simulink model "antiwindup_blockDiagram"  (R2025b)
settings: Solver=FixedStepAuto  StartTime=0.0  StopTime=5.0  FixedStep=0.01  RelTol=1e-3
model workspace (MAT data in the model file):
  Kawd = 1
  Ki = 1
  Kp = 1
values from neighbouring files (symbols this model uses):
  mu1 = 2.668    [StepResponseComparison.m]
  T1 = 0.47    [StepResponseComparison.m]
  Ts = time(2) - time(1)    [AntiwindupComparison.m]    (also in StepResponseComparison.m)
settings Model: Creator=favar  LastModifiedBy=favar

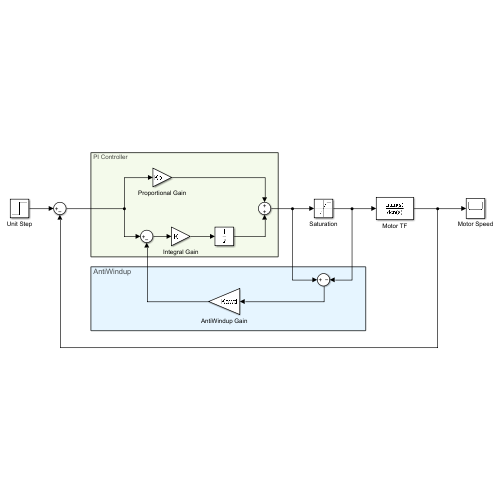
[thumbnail: Simulink's stored preview of the top-level diagram]
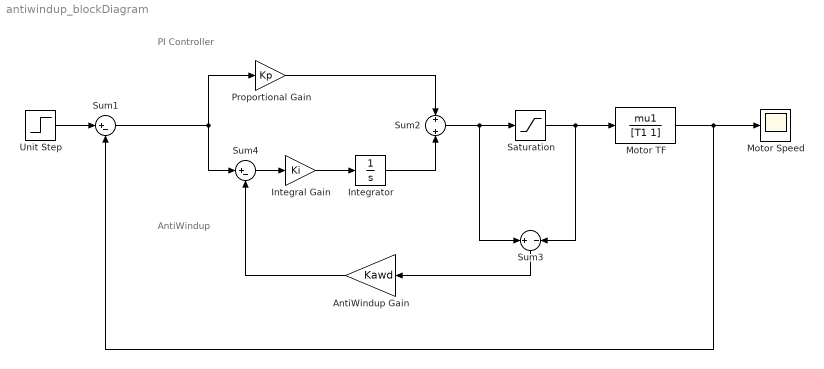
== system antiwindup_blockDiagram ==
  note: AntiWindup
  note: PI Controller
  AntiWindup Gain : Gain  Gain=Kawd
  Integral Gain : Gain  Gain=Ki
  Integrator : Integrator
  Motor Speed : Scope
  Motor TF : TransferFcn  Numerator=mu1  Denominator=[T1 1]
  Proportional Gain : Gain  Gain=Kp  RndMeth=Zero
  Saturation : Saturate
  Sum1 : Sum  Inputs=|+-
  Sum2 : Sum  Inputs=+||+
  Sum3 : Sum  Inputs=+||-
  Sum4 : Sum  Inputs=|+-
  Unit Step : Step  Time=Ts  After=10  SampleTime=0
  wires:
  Unit Step/1 -> Sum1/1
  Sum1/1 -> Sum4/1, Proportional Gain/1
  Proportional Gain/1 -> Sum2/1
  Integral Gain/1 -> Integrator/1
  Integrator/1 -> Sum2/2
  Sum2/1 -> Sum3/1, Saturation/1
  Saturation/1 -> Motor TF/1, Sum3/2
  Sum3/1 -> AntiWindup Gain/1
  Sum4/1 -> Integral Gain/1
  AntiWindup Gain/1 -> Sum4/2
  Motor TF/1 -> Sum1/2, Motor Speed/1
